simulink model "a4"  (R2018b)
settings: Solver=ode23tb  StartTime=0.0  StopTime=24*60*60  MaxStep=60  RelTol=1e-4
PreLoadFcn:
  | load('solar_load_data_24h.mat')
(part 2 of 2)

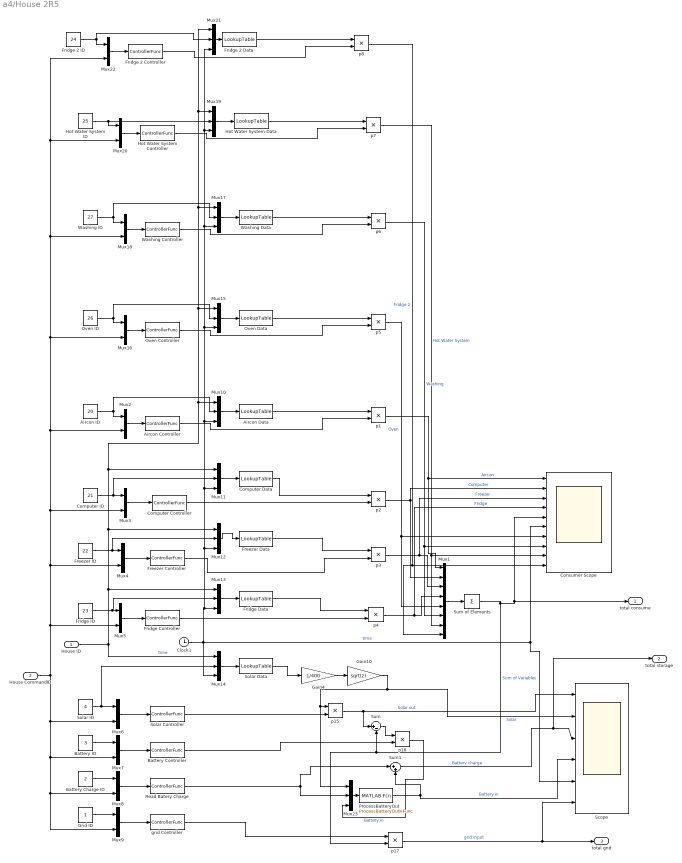
== system a4/House 2R5 ==
  House ID : Inport
  House CommandID : Inport  Port=2
  Aircon Controller : MATLABFcn  MATLABFcn=ControllerFunc  OutputSignalType=real
  Aircon Data : MATLABFcn  MATLABFcn=LookupTable  OutputSignalType=real
  Aircon ID : Constant  Value=20
  Battery Charge ID : Constant  Value=2
  Battery Controller : MATLABFcn  MATLABFcn=ControllerFunc  OutputSignalType=real
  Battery ID : Constant  Value=3
  Clock1 : Clock
  Computer Controller : MATLABFcn  MATLABFcn=ControllerFunc  OutputSignalType=real
  Computer Data : MATLABFcn  MATLABFcn=LookupTable  OutputSignalType=real
  Computer ID : Constant  Value=21
  Consumer Scope : Scope  NumInputPorts=10
  Freezer Controller : MATLABFcn  MATLABFcn=ControllerFunc  OutputSignalType=real
  Freezer Data : MATLABFcn  MATLABFcn=LookupTable  OutputSignalType=real
  Freezer ID : Constant  Value=22
  Fridge 2 Controller : MATLABFcn  MATLABFcn=ControllerFunc  OutputSignalType=real
  Fridge 2 Data : MATLABFcn  MATLABFcn=LookupTable  OutputSignalType=real
  Fridge 2 ID : Constant  Value=24
  Fridge Controller : MATLABFcn  MATLABFcn=ControllerFunc  OutputSignalType=real
  Fridge Data : MATLABFcn  MATLABFcn=LookupTable  OutputSignalType=real
  Fridge ID : Constant  Value=23
  Gain10 : Gain  Gain=sqrt(2)
  Gain4 : Gain  Gain=1/400
  Grid ID : Constant
  Hot Water System Controller : MATLABFcn  MATLABFcn=ControllerFunc  OutputSignalType=real
  Hot Water System Data : MATLABFcn  MATLABFcn=LookupTable  OutputSignalType=real
  Hot Water System ID : Constant  Value=25
  Mux1 : Mux  Inputs=8
  Mux{10..15,17,19,21,23} (10 alike) : Mux  Inputs=3
  Mux{2..9,16,18,20,22} (12 alike) : Mux  Inputs=2
  Oven Controller : MATLABFcn  MATLABFcn=ControllerFunc  OutputSignalType=real
  Oven Data : MATLABFcn  MATLABFcn=LookupTable  OutputSignalType=real
  Oven ID : Constant  Value=26
  ProcessBatteryOut : MATLABFcn  MATLABFcn=ProcessBatteryOutHFunc  OutputSignalType=real
  Read Batery Charge : MATLABFcn  MATLABFcn=ControllerFunc  OutputSignalType=real
  Scope : Scope  NumInputPorts=6
  Solar Controller : MATLABFcn  MATLABFcn=ControllerFunc  OutputSignalType=real
  Solar Data : MATLABFcn  MATLABFcn=LookupTable  OutputSignalType=real
  Solar ID : Constant  Value=4
  Sum : Sum  Inputs=|+-
  Sum of Elements : Sum  Inputs=+
  Sum1 : Sum  Inputs=|++
  Washing Controller : MATLABFcn  MATLABFcn=ControllerFunc  OutputSignalType=real
  Washing Data : MATLABFcn  MATLABFcn=LookupTable  OutputSignalType=real
  Washing ID : Constant  Value=27
  grid Controller : MATLABFcn  MATLABFcn=ControllerFunc  OutputSignalType=real
  p{1..8,15..17} (11 alike) : Product
  total consume : Outport
  total storage : Outport  Port=2
  total grid : Outport  Port=3
  wires:
  Clock1/1 -> Mux11/3, Mux21/3, Mux19/3, Mux17/3, Mux15/3, Mux10/3, Mux12/3, Mux13/3, Mux14/3, Scope/5, Consumer Scope/6  "time"
  Aircon Data/1 -> p1/1
  Mux1/1 -> Sum of Elements/1
  p1/1 -> Consumer Scope/1, Mux1/1  "Aircon"
  Sum of Elements/1 -> total consume/1, Consumer Scope/5, p17/2, Sum/2  "Sum of Variables"
  p4/1 -> Consumer Scope/4, Mux1/4  "Fridge"
  p2/1 -> Consumer Scope/2, Mux1/2  "Computer"
  p3/1 -> Consumer Scope/3, Mux1/3  "Freezer"
  Computer Controller/1 -> p2/2
  Freezer Controller/1 -> p3/2
  Solar Data/1 -> Gain4/1
  Solar Controller/1 -> p15/2
  Gain10/1 -> Scope/2, Mux23/1, p15/1  "Solar"
  p15/1 -> Sum/1, Scope/1  "Solar out"
  Sum/1 -> p16/1
  Battery Controller/1 -> p16/2
  Sum1/1 -> total storage/1, Scope/3  "Battery charge"
  grid Controller/1 -> p17/1
  p17/1 -> Scope/6, total grid/1  "grid input"
  Read Batery Charge/1 -> Mux23/2, Sum1/1
  p16/1 -> Mux23/3  "Battery in"
  ProcessBatteryOut/1 -> Scope/4, Sum1/2  "Battery in"
  Computer Data/1 -> p2/1
  Freezer Data/1 -> p3/1
  Fridge Data/1 -> p4/1
  Fridge Controller/1 -> p4/2
  Gain4/1 -> Gain10/1
  Aircon ID/1 -> Mux2/1, Mux10/2
  Computer ID/1 -> Mux11/2, Mux3/1
  Mux3/1 -> Computer Controller/1
  Freezer ID/1 -> Mux12/2, Mux4/1
  Mux4/1 -> Freezer Controller/1
  Mux5/1 -> Fridge Controller/1
  Fridge ID/1 -> Mux13/2, Mux5/1
  Mux6/1 -> Solar Controller/1
  Solar ID/1 -> Mux14/2, Mux6/1
  Mux7/1 -> Battery Controller/1
  Mux8/1 -> Read Batery Charge/1
  Mux9/1 -> grid Controller/1
  Battery ID/1 -> Mux7/1
  Battery Charge ID/1 -> Mux8/1
  Grid ID/1 -> Mux9/1
  Mux10/1 -> Aircon Data/1
  Mux11/1 -> Computer Data/1
  Mux12/1 -> Freezer Data/1
  Mux13/1 -> Fridge Data/1
  Mux14/1 -> Solar Data/1
  Aircon Controller/1 -> p1/2
  Mux2/1 -> Aircon Controller/1
  House CommandID/1 -> Mux9/2, Mux8/2, Mux7/2, Mux6/2, Mux3/2, Mux16/2, Mux20/2, Mux22/2, Mux18/2, Mux2/2, Mux4/2, Mux5/2
  Oven Data/1 -> p5/1
  Oven ID/1 -> Mux16/1, Mux15/2
  Mux15/1 -> Oven Data/1
  p5/1 -> Mux1/5, Consumer Scope/7  "Oven"
  Oven Controller/1 -> p5/2
  Washing Data/1 -> p6/1
  Washing ID/1 -> Mux18/1, Mux17/2
  Mux17/1 -> Washing Data/1
  p6/1 -> Mux1/6, Consumer Scope/8  "Washing"
  Washing Controller/1 -> p6/2
  Hot Water System Data/1 -> p7/1
  Hot Water System ID/1 -> Mux20/1, Mux19/2
  Mux19/1 -> Hot Water System Data/1
  p7/1 -> Mux1/7, Consumer Scope/9  "Hot Water System"
  Hot Water System Controller/1 -> p7/2
  Fridge 2 Data/1 -> p8/1
  Fridge 2 ID/1 -> Mux22/1, Mux21/2
  Mux21/1 -> Fridge 2 Data/1
  p8/1 -> Consumer Scope/10, Mux1/8  "Fridge 2"
  Fridge 2 Controller/1 -> p8/2
  House ID/1 -> Mux14/1, Mux21/1, Mux19/1, Mux17/1, Mux15/1, Mux10/1, Mux11/1, Mux12/1, Mux13/1  "time"
  Mux20/1 -> Hot Water System Controller/1
  Mux16/1 -> Oven Controller/1
  Mux18/1 -> Washing Controller/1
  Mux22/1 -> Fridge 2 Controller/1
  Mux23/1 -> ProcessBatteryOut/1

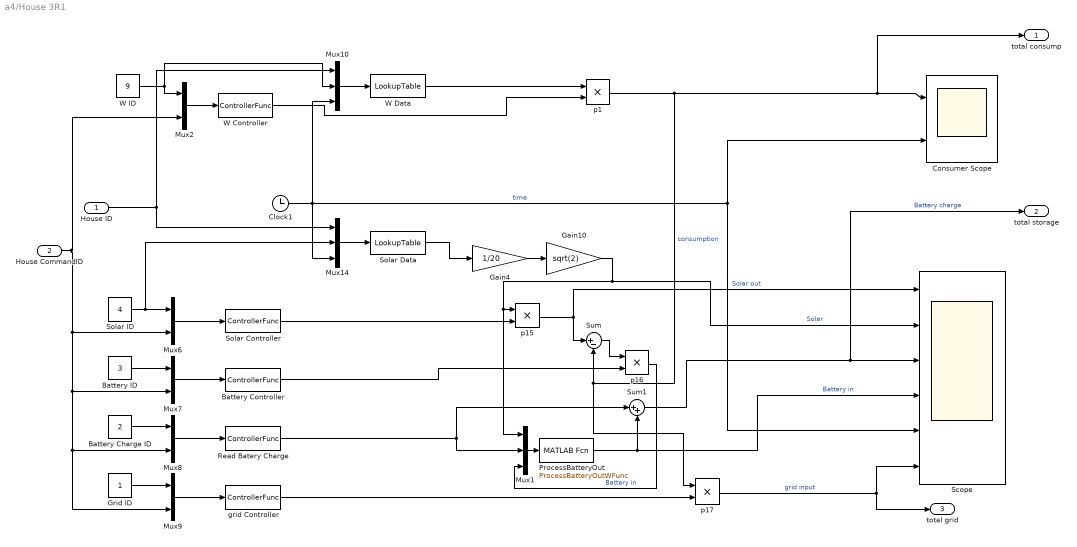
== system a4/House 3R1 ==
  House ID : Inport
  House CommandID : Inport  Port=2
  Battery Charge ID : Constant  Value=2
  Battery Controller : MATLABFcn  MATLABFcn=ControllerFunc  OutputSignalType=real
  Battery ID : Constant  Value=3
  Clock1 : Clock
  Consumer Scope : Scope  NumInputPorts=2
  Gain10 : Gain  Gain=sqrt(2)
  Gain4 : Gain  Gain=1/20
  Grid ID : Constant
  Mux1 : Mux  Inputs=3
  Mux10 : Mux  Inputs=3
  Mux14 : Mux  Inputs=3
  Mux{2,6..9} (5 alike) : Mux  Inputs=2
  ProcessBatteryOut : MATLABFcn  MATLABFcn=ProcessBatteryOutWFunc  OutputSignalType=real
  Read Batery Charge : MATLABFcn  MATLABFcn=ControllerFunc  OutputSignalType=real
  Scope : Scope  NumInputPorts=6
  Solar Controller : MATLABFcn  MATLABFcn=ControllerFunc  OutputSignalType=real
  Solar Data : MATLABFcn  MATLABFcn=LookupTable  OutputSignalType=real
  Solar ID : Constant  Value=4
  Sum : Sum  Inputs=|+-
  Sum1 : Sum  Inputs=|++
  W Controller : MATLABFcn  MATLABFcn=ControllerFunc  OutputSignalType=real
  W Data : MATLABFcn  MATLABFcn=LookupTable  OutputSignalType=real
  W ID : Constant  Value=9
  grid Controller : MATLABFcn  MATLABFcn=ControllerFunc  OutputSignalType=real
  p{1,15..17} (4 alike) : Product
  total consump : Outport
  total storage : Outport  Port=2
  total grid : Outport  Port=3
  wires:
  Clock1/1 -> Mux10/3, Mux14/3, Scope/5, Consumer Scope/2  "time"
  W Data/1 -> p1/1
  Solar Data/1 -> Gain4/1
  Solar Controller/1 -> p15/2
  Gain10/1 -> Scope/2, Mux1/1, p15/1  "Solar"
  p15/1 -> Sum/1, Scope/1  "Solar out"
  Sum/1 -> p16/1
  Battery Controller/1 -> p16/2
  Sum1/1 -> total storage/1, Scope/3  "Battery charge"
  grid Controller/1 -> p17/2
  p17/1 -> Scope/6, total grid/1  "grid input"
  Read Batery Charge/1 -> Sum1/1, Mux1/2
  p16/1 -> Mux1/3  "Battery in"
  ProcessBatteryOut/1 -> Scope/4, Sum1/2  "Battery in"
  Mux1/1 -> ProcessBatteryOut/1
  Gain4/1 -> Gain10/1
  W ID/1 -> Mux2/1, Mux10/2
  House ID/1 -> Mux10/1, Mux14/1
  Mux6/1 -> Solar Controller/1
  Solar ID/1 -> Mux14/2, Mux6/1
  Mux7/1 -> Battery Controller/1
  Mux8/1 -> Read Batery Charge/1
  Mux9/1 -> grid Controller/1
  Battery ID/1 -> Mux7/1
  Battery Charge ID/1 -> Mux8/1
  Grid ID/1 -> Mux9/1
  Mux10/1 -> W Data/1
  Mux14/1 -> Solar Data/1
  W Controller/1 -> p1/2
  Mux2/1 -> W Controller/1
  p1/1 -> p17/1, Sum/2, total consump/1, Consumer Scope/1  "consumption"
  House CommandID/1 -> Mux9/2, Mux8/2, Mux7/2, Mux6/2, Mux2/2

== system a4/House 3R2 ==
  House ID : Inport
  House CommandID : Inport  Port=2
  Battery Charge ID : Constant  Value=2
  Battery Controller : MATLABFcn  MATLABFcn=ControllerFunc  OutputSignalType=real
  Battery ID : Constant  Value=3
  Clock1 : Clock
  Consumer Scope : Scope  NumInputPorts=2
  Gain10 : Gain  Gain=sqrt(2)
  Gain4 : Gain  Gain=1/20
  Grid ID : Constant
  Mux1 : Mux  Inputs=3
  Mux10 : Mux  Inputs=3
  Mux14 : Mux  Inputs=3
  Mux{2,6..9} (5 alike) : Mux  Inputs=2
  ProcessBatteryOut : MATLABFcn  MATLABFcn=ProcessBatteryOutWFunc  OutputSignalType=real
  Read Batery Charge : MATLABFcn  MATLABFcn=ControllerFunc  OutputSignalType=real
  Scope : Scope  NumInputPorts=6
  Solar Controller : MATLABFcn  MATLABFcn=ControllerFunc  OutputSignalType=real
  Solar Data : MATLABFcn  MATLABFcn=LookupTable  OutputSignalType=real
  Solar ID : Constant  Value=4
  Sum : Sum  Inputs=|+-
  Sum1 : Sum  Inputs=|++
  W Controller : MATLABFcn  MATLABFcn=ControllerFunc  OutputSignalType=real
  W Data : MATLABFcn  MATLABFcn=LookupTable  OutputSignalType=real
  W ID : Constant  Value=9
  grid Controller : MATLABFcn  MATLABFcn=ControllerFunc  OutputSignalType=real
  p{1,15..17} (4 alike) : Product
  total consump : Outport
  total storage : Outport  Port=2
  total grid : Outport  Port=3
  wires:
  House CommandID/1 -> Mux2/2, Mux6/2, Mux7/2, Mux8/2, Mux9/2
  p1/1 -> Consumer Scope/1, total consump/1, Sum/2, p17/1  "consumption"
  Mux2/1 -> W Controller/1
  W Controller/1 -> p1/2
  Mux14/1 -> Solar Data/1
  Mux10/1 -> W Data/1
  Grid ID/1 -> Mux9/1
  Battery Charge ID/1 -> Mux8/1
  Battery ID/1 -> Mux7/1
  Mux9/1 -> grid Controller/1
  Mux8/1 -> Read Batery Charge/1
  Mux7/1 -> Battery Controller/1
  Solar ID/1 -> Mux6/1, Mux14/2
  Mux6/1 -> Solar Controller/1
  House ID/1 -> Mux14/1, Mux10/1
  W ID/1 -> Mux10/2, Mux2/1
  Gain4/1 -> Gain10/1
  Mux1/1 -> ProcessBatteryOut/1
  ProcessBatteryOut/1 -> Sum1/2, Scope/4  "Battery in"
  p16/1 -> Mux1/3  "Battery in"
  Read Batery Charge/1 -> Mux1/2, Sum1/1
  p17/1 -> total grid/1, Scope/6  "grid input"
  grid Controller/1 -> p17/2
  Sum1/1 -> Scope/3, total storage/1  "Battery charge"
  Battery Controller/1 -> p16/2
  Sum/1 -> p16/1
  p15/1 -> Scope/1, Sum/1  "Solar out"
  Gain10/1 -> p15/1, Mux1/1, Scope/2  "Solar"
  Solar Controller/1 -> p15/2
  Solar Data/1 -> Gain4/1
  W Data/1 -> p1/1
  Clock1/1 -> Consumer Scope/2, Scope/5, Mux14/3, Mux10/3  "time"

== system a4/House 3R3 ==
  House ID : Inport
  House CommandID : Inport  Port=2
  Battery Charge ID : Constant  Value=2
  Battery Controller : MATLABFcn  MATLABFcn=ControllerFunc  OutputSignalType=real
  Battery ID : Constant  Value=3
  Clock1 : Clock
  Consumer Scope : Scope  NumInputPorts=2
  Gain10 : Gain  Gain=sqrt(2)
  Gain4 : Gain  Gain=1/20
  Grid ID : Constant
  Mux1 : Mux  Inputs=3
  Mux10 : Mux  Inputs=3
  Mux14 : Mux  Inputs=3
  Mux{2,6..9} (5 alike) : Mux  Inputs=2
  ProcessBatteryOut : MATLABFcn  MATLABFcn=ProcessBatteryOutWFunc  OutputSignalType=real
  Read Batery Charge : MATLABFcn  MATLABFcn=ControllerFunc  OutputSignalType=real
  Scope : Scope  NumInputPorts=6
  Solar Controller : MATLABFcn  MATLABFcn=ControllerFunc  OutputSignalType=real
  Solar Data : MATLABFcn  MATLABFcn=LookupTable  OutputSignalType=real
  Solar ID : Constant  Value=4
  Sum : Sum  Inputs=|+-
  Sum1 : Sum  Inputs=|++
  W Controller : MATLABFcn  MATLABFcn=ControllerFunc  OutputSignalType=real
  W Data : MATLABFcn  MATLABFcn=LookupTable  OutputSignalType=real
  W ID : Constant  Value=9
  grid Controller : MATLABFcn  MATLABFcn=ControllerFunc  OutputSignalType=real
  p{1,15..17} (4 alike) : Product
  total consump : Outport
  total storage : Outport  Port=2
  total grid : Outport  Port=3
  wires:
  Clock1/1 -> Mux10/3, Mux14/3, Scope/5, Consumer Scope/2  "time"
  W Data/1 -> p1/1
  Solar Data/1 -> Gain4/1
  Solar Controller/1 -> p15/2
  Gain10/1 -> Scope/2, Mux1/1, p15/1  "Solar"
  p15/1 -> Sum/1, Scope/1  "Solar out"
  Sum/1 -> p16/1
  Battery Controller/1 -> p16/2
  Sum1/1 -> total storage/1, Scope/3  "Battery charge"
  grid Controller/1 -> p17/2
  p17/1 -> Scope/6, total grid/1  "grid input"
  Read Batery Charge/1 -> Sum1/1, Mux1/2
  p16/1 -> Mux1/3  "Battery in"
  ProcessBatteryOut/1 -> Scope/4, Sum1/2  "Battery in"
  Mux1/1 -> ProcessBatteryOut/1
  Gain4/1 -> Gain10/1
  W ID/1 -> Mux2/1, Mux10/2
  House ID/1 -> Mux10/1, Mux14/1
  Mux6/1 -> Solar Controller/1
  Solar ID/1 -> Mux14/2, Mux6/1
  Mux7/1 -> Battery Controller/1
  Mux8/1 -> Read Batery Charge/1
  Mux9/1 -> grid Controller/1
  Battery ID/1 -> Mux7/1
  Battery Charge ID/1 -> Mux8/1
  Grid ID/1 -> Mux9/1
  Mux10/1 -> W Data/1
  Mux14/1 -> Solar Data/1
  W Controller/1 -> p1/2
  Mux2/1 -> W Controller/1
  p1/1 -> p17/1, Sum/2, total consump/1, Consumer Scope/1  "consumption"
  House CommandID/1 -> Mux9/2, Mux8/2, Mux7/2, Mux6/2, Mux2/2

== system a4/House 3R4 ==
  House ID : Inport
  House CommandID : Inport  Port=2
  Battery Charge ID : Constant  Value=2
  Battery Controller : MATLABFcn  MATLABFcn=ControllerFunc  OutputSignalType=real
  Battery ID : Constant  Value=3
  Clock1 : Clock
  Consumer Scope : Scope  NumInputPorts=2
  Gain10 : Gain  Gain=sqrt(2)
  Gain4 : Gain  Gain=1/20
  Grid ID : Constant
  Mux1 : Mux  Inputs=3
  Mux10 : Mux  Inputs=3
  Mux14 : Mux  Inputs=3
  Mux{2,6..9} (5 alike) : Mux  Inputs=2
  ProcessBatteryOut : MATLABFcn  MATLABFcn=ProcessBatteryOutWFunc  OutputSignalType=real
  Read Batery Charge : MATLABFcn  MATLABFcn=ControllerFunc  OutputSignalType=real
  Scope : Scope  NumInputPorts=6
  Solar Controller : MATLABFcn  MATLABFcn=ControllerFunc  OutputSignalType=real
  Solar Data : MATLABFcn  MATLABFcn=LookupTable  OutputSignalType=real
  Solar ID : Constant  Value=4
  Sum : Sum  Inputs=|+-
  Sum1 : Sum  Inputs=|++
  W Controller : MATLABFcn  MATLABFcn=ControllerFunc  OutputSignalType=real
  W Data : MATLABFcn  MATLABFcn=LookupTable  OutputSignalType=real
  W ID : Constant  Value=9
  grid Controller : MATLABFcn  MATLABFcn=ControllerFunc  OutputSignalType=real
  p{1,15..17} (4 alike) : Product
  total consump : Outport
  total storage : Outport  Port=2
  total grid : Outport  Port=3
  wires:
  House CommandID/1 -> Mux2/2, Mux6/2, Mux7/2, Mux8/2, Mux9/2
  p1/1 -> Consumer Scope/1, total consump/1, Sum/2, p17/1  "consumption"
  Mux2/1 -> W Controller/1
  W Controller/1 -> p1/2
  Mux14/1 -> Solar Data/1
  Mux10/1 -> W Data/1
  Grid ID/1 -> Mux9/1
  Battery Charge ID/1 -> Mux8/1
  Battery ID/1 -> Mux7/1
  Mux9/1 -> grid Controller/1
  Mux8/1 -> Read Batery Charge/1
  Mux7/1 -> Battery Controller/1
  Solar ID/1 -> Mux6/1, Mux14/2
  Mux6/1 -> Solar Controller/1
  House ID/1 -> Mux14/1, Mux10/1
  W ID/1 -> Mux10/2, Mux2/1
  Gain4/1 -> Gain10/1
  Mux1/1 -> ProcessBatteryOut/1
  ProcessBatteryOut/1 -> Sum1/2, Scope/4  "Battery in"
  p16/1 -> Mux1/3  "Battery in"
  Read Batery Charge/1 -> Mux1/2, Sum1/1
  p17/1 -> total grid/1, Scope/6  "grid input"
  grid Controller/1 -> p17/2
  Sum1/1 -> Scope/3, total storage/1  "Battery charge"
  Battery Controller/1 -> p16/2
  Sum/1 -> p16/1
  p15/1 -> Scope/1, Sum/1  "Solar out"
  Gain10/1 -> p15/1, Mux1/1, Scope/2  "Solar"
  Solar Controller/1 -> p15/2
  Solar Data/1 -> Gain4/1
  W Data/1 -> p1/1
  Clock1/1 -> Consumer Scope/2, Scope/5, Mux14/3, Mux10/3  "time"

== system a4/House 3R5 ==
  House ID : Inport
  House CommandID : Inport  Port=2
  Battery Charge ID : Constant  Value=2
  Battery Controller : MATLABFcn  MATLABFcn=ControllerFunc  OutputSignalType=real
  Battery ID : Constant  Value=3
  Clock1 : Clock
  Consumer Scope : Scope  NumInputPorts=2
  Gain10 : Gain  Gain=sqrt(2)
  Gain4 : Gain  Gain=1/20
  Grid ID : Constant
  Mux1 : Mux  Inputs=3
  Mux10 : Mux  Inputs=3
  Mux14 : Mux  Inputs=3
  Mux{2,6..9} (5 alike) : Mux  Inputs=2
  ProcessBatteryOut : MATLABFcn  MATLABFcn=ProcessBatteryOutWFunc  OutputSignalType=real
  Read Batery Charge : MATLABFcn  MATLABFcn=ControllerFunc  OutputSignalType=real
  Scope : Scope  NumInputPorts=6
  Solar Controller : MATLABFcn  MATLABFcn=ControllerFunc  OutputSignalType=real
  Solar Data : MATLABFcn  MATLABFcn=LookupTable  OutputSignalType=real
  Solar ID : Constant  Value=4
  Sum : Sum  Inputs=|+-
  Sum1 : Sum  Inputs=|++
  W Controller : MATLABFcn  MATLABFcn=ControllerFunc  OutputSignalType=real
  W Data : MATLABFcn  MATLABFcn=LookupTable  OutputSignalType=real
  W ID : Constant  Value=9
  grid Controller : MATLABFcn  MATLABFcn=ControllerFunc  OutputSignalType=real
  p{1,15..17} (4 alike) : Product
  total consump : Outport
  total storage : Outport  Port=2
  total grid : Outport  Port=3
  wires:
  Clock1/1 -> Mux10/3, Mux14/3, Scope/5, Consumer Scope/2  "time"
  W Data/1 -> p1/1
  Solar Data/1 -> Gain4/1
  Solar Controller/1 -> p15/2
  Gain10/1 -> Scope/2, Mux1/1, p15/1  "Solar"
  p15/1 -> Sum/1, Scope/1  "Solar out"
  Sum/1 -> p16/1
  Battery Controller/1 -> p16/2
  Sum1/1 -> total storage/1, Scope/3  "Battery charge"
  grid Controller/1 -> p17/2
  p17/1 -> Scope/6, total grid/1  "grid input"
  Read Batery Charge/1 -> Sum1/1, Mux1/2
  p16/1 -> Mux1/3  "Battery in"
  ProcessBatteryOut/1 -> Scope/4, Sum1/2  "Battery in"
  Mux1/1 -> ProcessBatteryOut/1
  Gain4/1 -> Gain10/1
  W ID/1 -> Mux2/1, Mux10/2
  House ID/1 -> Mux10/1, Mux14/1
  Mux6/1 -> Solar Controller/1
  Solar ID/1 -> Mux14/2, Mux6/1
  Mux7/1 -> Battery Controller/1
  Mux8/1 -> Read Batery Charge/1
  Mux9/1 -> grid Controller/1
  Battery ID/1 -> Mux7/1
  Battery Charge ID/1 -> Mux8/1
  Grid ID/1 -> Mux9/1
  Mux10/1 -> W Data/1
  Mux14/1 -> Solar Data/1
  W Controller/1 -> p1/2
  Mux2/1 -> W Controller/1
  p1/1 -> p17/1, Sum/2, total consump/1, Consumer Scope/1  "consumption"
  House CommandID/1 -> Mux9/2, Mux8/2, Mux7/2, Mux6/2, Mux2/2

== system a4/House 4R1 ==
  House ID : Inport
  House CommandID : Inport  Port=2
  Battery Charge ID : Constant  Value=2
  Battery Controller : MATLABFcn  MATLABFcn=ControllerFunc  OutputSignalType=real
  Battery ID : Constant  Value=3
  Clock1 : Clock
  Consumer Scope : Scope  NumInputPorts=2
  Gain10 : Gain  Gain=sqrt(2)
  Gain4 : Gain  Gain=1/20
  Grid ID : Constant
  Mux1 : Mux  Inputs=3
  Mux10 : Mux  Inputs=3
  Mux14 : Mux  Inputs=3
  Mux{2,6..9} (5 alike) : Mux  Inputs=2
  ProcessBatteryOut : MATLABFcn  MATLABFcn=ProcessBatteryOutWFunc  OutputSignalType=real
  Read Batery Charge : MATLABFcn  MATLABFcn=ControllerFunc  OutputSignalType=real
  Scope : Scope  NumInputPorts=6
  Solar Controller : MATLABFcn  MATLABFcn=ControllerFunc  OutputSignalType=real
  Solar Data : MATLABFcn  MATLABFcn=LookupTable  OutputSignalType=real
  Solar ID : Constant  Value=4
  Sum : Sum  Inputs=|+-
  Sum1 : Sum  Inputs=|++
  W Controller : MATLABFcn  MATLABFcn=ControllerFunc  OutputSignalType=real
  W Data : MATLABFcn  MATLABFcn=LookupTable  OutputSignalType=real
  W ID : Constant  Value=9
  grid Controller : MATLABFcn  MATLABFcn=ControllerFunc  OutputSignalType=real
  p{1,15..17} (4 alike) : Product
  total consump : Outport
  total storage : Outport  Port=2
  total grid : Outport  Port=3
  wires:
  House CommandID/1 -> Mux2/2, Mux6/2, Mux7/2, Mux8/2, Mux9/2
  p1/1 -> Consumer Scope/1, total consump/1, Sum/2, p17/1  "consumption"
  Mux2/1 -> W Controller/1
  W Controller/1 -> p1/2
  Mux14/1 -> Solar Data/1
  Mux10/1 -> W Data/1
  Grid ID/1 -> Mux9/1
  Battery Charge ID/1 -> Mux8/1
  Battery ID/1 -> Mux7/1
  Mux9/1 -> grid Controller/1
  Mux8/1 -> Read Batery Charge/1
  Mux7/1 -> Battery Controller/1
  Solar ID/1 -> Mux6/1, Mux14/2
  Mux6/1 -> Solar Controller/1
  House ID/1 -> Mux14/1, Mux10/1
  W ID/1 -> Mux10/2, Mux2/1
  Gain4/1 -> Gain10/1
  Mux1/1 -> ProcessBatteryOut/1
  ProcessBatteryOut/1 -> Sum1/2, Scope/4  "Battery in"
  p16/1 -> Mux1/3  "Battery in"
  Read Batery Charge/1 -> Mux1/2, Sum1/1
  p17/1 -> total grid/1, Scope/6  "grid input"
  grid Controller/1 -> p17/2
  Sum1/1 -> Scope/3, total storage/1  "Battery charge"
  Battery Controller/1 -> p16/2
  Sum/1 -> p16/1
  p15/1 -> Scope/1, Sum/1  "Solar out"
  Gain10/1 -> p15/1, Mux1/1, Scope/2  "Solar"
  Solar Controller/1 -> p15/2
  Solar Data/1 -> Gain4/1
  W Data/1 -> p1/1
  Clock1/1 -> Consumer Scope/2, Scope/5, Mux14/3, Mux10/3  "time"

== system a4/House 4R2 ==
  House ID : Inport
  House CommandID : Inport  Port=2
  Battery Charge ID : Constant  Value=2
  Battery Controller : MATLABFcn  MATLABFcn=ControllerFunc  OutputSignalType=real
  Battery ID : Constant  Value=3
  Clock1 : Clock
  Consumer Scope : Scope  NumInputPorts=2
  Gain10 : Gain  Gain=sqrt(2)
  Gain4 : Gain  Gain=1/20
  Grid ID : Constant
  Mux1 : Mux  Inputs=3
  Mux10 : Mux  Inputs=3
  Mux14 : Mux  Inputs=3
  Mux{2,6..9} (5 alike) : Mux  Inputs=2
  ProcessBatteryOut : MATLABFcn  MATLABFcn=ProcessBatteryOutWFunc  OutputSignalType=real
  Read Batery Charge : MATLABFcn  MATLABFcn=ControllerFunc  OutputSignalType=real
  Scope : Scope  NumInputPorts=6
  Solar Controller : MATLABFcn  MATLABFcn=ControllerFunc  OutputSignalType=real
  Solar Data : MATLABFcn  MATLABFcn=LookupTable  OutputSignalType=real
  Solar ID : Constant  Value=4
  Sum : Sum  Inputs=|+-
  Sum1 : Sum  Inputs=|++
  W Controller : MATLABFcn  MATLABFcn=ControllerFunc  OutputSignalType=real
  W Data : MATLABFcn  MATLABFcn=LookupTable  OutputSignalType=real
  W ID : Constant  Value=9
  grid Controller : MATLABFcn  MATLABFcn=ControllerFunc  OutputSignalType=real
  p{1,15..17} (4 alike) : Product
  total consump : Outport
  total storage : Outport  Port=2
  total grid : Outport  Port=3
  wires:
  Clock1/1 -> Mux10/3, Mux14/3, Scope/5, Consumer Scope/2  "time"
  W Data/1 -> p1/1
  Solar Data/1 -> Gain4/1
  Solar Controller/1 -> p15/2
  Gain10/1 -> Scope/2, Mux1/1, p15/1  "Solar"
  p15/1 -> Sum/1, Scope/1  "Solar out"
  Sum/1 -> p16/1
  Battery Controller/1 -> p16/2
  Sum1/1 -> total storage/1, Scope/3  "Battery charge"
  grid Controller/1 -> p17/2
  p17/1 -> Scope/6, total grid/1  "grid input"
  Read Batery Charge/1 -> Sum1/1, Mux1/2
  p16/1 -> Mux1/3  "Battery in"
  ProcessBatteryOut/1 -> Scope/4, Sum1/2  "Battery in"
  Mux1/1 -> ProcessBatteryOut/1
  Gain4/1 -> Gain10/1
  W ID/1 -> Mux2/1, Mux10/2
  House ID/1 -> Mux10/1, Mux14/1
  Mux6/1 -> Solar Controller/1
  Solar ID/1 -> Mux14/2, Mux6/1
  Mux7/1 -> Battery Controller/1
  Mux8/1 -> Read Batery Charge/1
  Mux9/1 -> grid Controller/1
  Battery ID/1 -> Mux7/1
  Battery Charge ID/1 -> Mux8/1
  Grid ID/1 -> Mux9/1
  Mux10/1 -> W Data/1
  Mux14/1 -> Solar Data/1
  W Controller/1 -> p1/2
  Mux2/1 -> W Controller/1
  p1/1 -> p17/1, Sum/2, total consump/1, Consumer Scope/1  "consumption"
  House CommandID/1 -> Mux9/2, Mux8/2, Mux7/2, Mux6/2, Mux2/2

== system a4/House 4R3 ==
  House ID : Inport
  House CommandID : Inport  Port=2
  Battery Charge ID : Constant  Value=2
  Battery Controller : MATLABFcn  MATLABFcn=ControllerFunc  OutputSignalType=real
  Battery ID : Constant  Value=3
  Clock1 : Clock
  Consumer Scope : Scope  NumInputPorts=2
  Gain10 : Gain  Gain=sqrt(2)
  Gain4 : Gain  Gain=1/20
  Grid ID : Constant
  Mux1 : Mux  Inputs=3
  Mux10 : Mux  Inputs=3
  Mux14 : Mux  Inputs=3
  Mux{2,6..9} (5 alike) : Mux  Inputs=2
  ProcessBatteryOut : MATLABFcn  MATLABFcn=ProcessBatteryOutWFunc  OutputSignalType=real
  Read Batery Charge : MATLABFcn  MATLABFcn=ControllerFunc  OutputSignalType=real
  Scope : Scope  NumInputPorts=6
  Solar Controller : MATLABFcn  MATLABFcn=ControllerFunc  OutputSignalType=real
  Solar Data : MATLABFcn  MATLABFcn=LookupTable  OutputSignalType=real
  Solar ID : Constant  Value=4
  Sum : Sum  Inputs=|+-
  Sum1 : Sum  Inputs=|++
  W Controller : MATLABFcn  MATLABFcn=ControllerFunc  OutputSignalType=real
  W Data : MATLABFcn  MATLABFcn=LookupTable  OutputSignalType=real
  W ID : Constant  Value=9
  grid Controller : MATLABFcn  MATLABFcn=ControllerFunc  OutputSignalType=real
  p{1,15..17} (4 alike) : Product
  total consump : Outport
  total storage : Outport  Port=2
  total grid : Outport  Port=3
  wires:
  House CommandID/1 -> Mux2/2, Mux6/2, Mux7/2, Mux8/2, Mux9/2
  p1/1 -> Consumer Scope/1, total consump/1, Sum/2, p17/1  "consumption"
  Mux2/1 -> W Controller/1
  W Controller/1 -> p1/2
  Mux14/1 -> Solar Data/1
  Mux10/1 -> W Data/1
  Grid ID/1 -> Mux9/1
  Battery Charge ID/1 -> Mux8/1
  Battery ID/1 -> Mux7/1
  Mux9/1 -> grid Controller/1
  Mux8/1 -> Read Batery Charge/1
  Mux7/1 -> Battery Controller/1
  Solar ID/1 -> Mux6/1, Mux14/2
  Mux6/1 -> Solar Controller/1
  House ID/1 -> Mux14/1, Mux10/1
  W ID/1 -> Mux10/2, Mux2/1
  Gain4/1 -> Gain10/1
  Mux1/1 -> ProcessBatteryOut/1
  ProcessBatteryOut/1 -> Sum1/2, Scope/4  "Battery in"
  p16/1 -> Mux1/3  "Battery in"
  Read Batery Charge/1 -> Mux1/2, Sum1/1
  p17/1 -> total grid/1, Scope/6  "grid input"
  grid Controller/1 -> p17/2
  Sum1/1 -> Scope/3, total storage/1  "Battery charge"
  Battery Controller/1 -> p16/2
  Sum/1 -> p16/1
  p15/1 -> Scope/1, Sum/1  "Solar out"
  Gain10/1 -> p15/1, Mux1/1, Scope/2  "Solar"
  Solar Controller/1 -> p15/2
  Solar Data/1 -> Gain4/1
  W Data/1 -> p1/1
  Clock1/1 -> Consumer Scope/2, Scope/5, Mux14/3, Mux10/3  "time"

== system a4/House 4R4 ==
  House ID : Inport
  House CommandID : Inport  Port=2
  Battery Charge ID : Constant  Value=2
  Battery Controller : MATLABFcn  MATLABFcn=ControllerFunc  OutputSignalType=real
  Battery ID : Constant  Value=3
  Clock1 : Clock
  Consumer Scope : Scope  NumInputPorts=2
  Gain10 : Gain  Gain=sqrt(2)
  Gain4 : Gain  Gain=1/20
  Grid ID : Constant
  Mux1 : Mux  Inputs=3
  Mux10 : Mux  Inputs=3
  Mux14 : Mux  Inputs=3
  Mux{2,6..9} (5 alike) : Mux  Inputs=2
  ProcessBatteryOut : MATLABFcn  MATLABFcn=ProcessBatteryOutWFunc  OutputSignalType=real
  Read Batery Charge : MATLABFcn  MATLABFcn=ControllerFunc  OutputSignalType=real
  Scope : Scope  NumInputPorts=6
  Solar Controller : MATLABFcn  MATLABFcn=ControllerFunc  OutputSignalType=real
  Solar Data : MATLABFcn  MATLABFcn=LookupTable  OutputSignalType=real
  Solar ID : Constant  Value=4
  Sum : Sum  Inputs=|+-
  Sum1 : Sum  Inputs=|++
  W Controller : MATLABFcn  MATLABFcn=ControllerFunc  OutputSignalType=real
  W Data : MATLABFcn  MATLABFcn=LookupTable  OutputSignalType=real
  W ID : Constant  Value=9
  grid Controller : MATLABFcn  MATLABFcn=ControllerFunc  OutputSignalType=real
  p{1,15..17} (4 alike) : Product
  total consump : Outport
  total storage : Outport  Port=2
  total grid : Outport  Port=3
  wires:
  Clock1/1 -> Mux10/3, Mux14/3, Scope/5, Consumer Scope/2  "time"
  W Data/1 -> p1/1
  Solar Data/1 -> Gain4/1
  Solar Controller/1 -> p15/2
  Gain10/1 -> Scope/2, Mux1/1, p15/1  "Solar"
  p15/1 -> Sum/1, Scope/1  "Solar out"
  Sum/1 -> p16/1
  Battery Controller/1 -> p16/2
  Sum1/1 -> total storage/1, Scope/3  "Battery charge"
  grid Controller/1 -> p17/2
  p17/1 -> Scope/6, total grid/1  "grid input"
  Read Batery Charge/1 -> Sum1/1, Mux1/2
  p16/1 -> Mux1/3  "Battery in"
  ProcessBatteryOut/1 -> Scope/4, Sum1/2  "Battery in"
  Mux1/1 -> ProcessBatteryOut/1
  Gain4/1 -> Gain10/1
  W ID/1 -> Mux2/1, Mux10/2
  House ID/1 -> Mux10/1, Mux14/1
  Mux6/1 -> Solar Controller/1
  Solar ID/1 -> Mux14/2, Mux6/1
  Mux7/1 -> Battery Controller/1
  Mux8/1 -> Read Batery Charge/1
  Mux9/1 -> grid Controller/1
  Battery ID/1 -> Mux7/1
  Battery Charge ID/1 -> Mux8/1
  Grid ID/1 -> Mux9/1
  Mux10/1 -> W Data/1
  Mux14/1 -> Solar Data/1
  W Controller/1 -> p1/2
  Mux2/1 -> W Controller/1
  p1/1 -> p17/1, Sum/2, total consump/1, Consumer Scope/1  "consumption"
  House CommandID/1 -> Mux9/2, Mux8/2, Mux7/2, Mux6/2, Mux2/2

== system a4/House 4R5 ==
  House ID : Inport
  House CommandID : Inport  Port=2
  Battery Charge ID : Constant  Value=2
  Battery Controller : MATLABFcn  MATLABFcn=ControllerFunc  OutputSignalType=real
  Battery ID : Constant  Value=3
  Clock1 : Clock
  Consumer Scope : Scope  NumInputPorts=2
  Gain10 : Gain  Gain=sqrt(2)
  Gain4 : Gain  Gain=1/20
  Grid ID : Constant
  Mux1 : Mux  Inputs=3
  Mux10 : Mux  Inputs=3
  Mux14 : Mux  Inputs=3
  Mux{2,6..9} (5 alike) : Mux  Inputs=2
  ProcessBatteryOut : MATLABFcn  MATLABFcn=ProcessBatteryOutWFunc  OutputSignalType=real
  Read Batery Charge : MATLABFcn  MATLABFcn=ControllerFunc  OutputSignalType=real
  Scope : Scope  NumInputPorts=6
  Solar Controller : MATLABFcn  MATLABFcn=ControllerFunc  OutputSignalType=real
  Solar Data : MATLABFcn  MATLABFcn=LookupTable  OutputSignalType=real
  Solar ID : Constant  Value=4
  Sum : Sum  Inputs=|+-
  Sum1 : Sum  Inputs=|++
  W Controller : MATLABFcn  MATLABFcn=ControllerFunc  OutputSignalType=real
  W Data : MATLABFcn  MATLABFcn=LookupTable  OutputSignalType=real
  W ID : Constant  Value=9
  grid Controller : MATLABFcn  MATLABFcn=ControllerFunc  OutputSignalType=real
  p{1,15..17} (4 alike) : Product
  total consump : Outport
  total storage : Outport  Port=2
  total grid : Outport  Port=3
  wires:
  House CommandID/1 -> Mux2/2, Mux6/2, Mux7/2, Mux8/2, Mux9/2
  p1/1 -> Consumer Scope/1, total consump/1, Sum/2, p17/1  "consumption"
  Mux2/1 -> W Controller/1
  W Controller/1 -> p1/2
  Mux14/1 -> Solar Data/1
  Mux10/1 -> W Data/1
  Grid ID/1 -> Mux9/1
  Battery Charge ID/1 -> Mux8/1
  Battery ID/1 -> Mux7/1
  Mux9/1 -> grid Controller/1
  Mux8/1 -> Read Batery Charge/1
  Mux7/1 -> Battery Controller/1
  Solar ID/1 -> Mux6/1, Mux14/2
  Mux6/1 -> Solar Controller/1
  House ID/1 -> Mux14/1, Mux10/1
  W ID/1 -> Mux10/2, Mux2/1
  Gain4/1 -> Gain10/1
  Mux1/1 -> ProcessBatteryOut/1
  ProcessBatteryOut/1 -> Sum1/2, Scope/4  "Battery in"
  p16/1 -> Mux1/3  "Battery in"
  Read Batery Charge/1 -> Mux1/2, Sum1/1
  p17/1 -> total grid/1, Scope/6  "grid input"
  grid Controller/1 -> p17/2
  Sum1/1 -> Scope/3, total storage/1  "Battery charge"
  Battery Controller/1 -> p16/2
  Sum/1 -> p16/1
  p15/1 -> Scope/1, Sum/1  "Solar out"
  Gain10/1 -> p15/1, Mux1/1, Scope/2  "Solar"
  Solar Controller/1 -> p15/2
  Solar Data/1 -> Gain4/1
  W Data/1 -> p1/1
  Clock1/1 -> Consumer Scope/2, Scope/5, Mux14/3, Mux10/3  "time"

== system a4/House 5R1 ==
  House ID : Inport
  House CommandID : Inport  Port=2
  Battery Charge ID : Constant  Value=2
  Battery Controller : MATLABFcn  MATLABFcn=ControllerFunc  OutputSignalType=real
  Battery ID : Constant  Value=3
  Clock1 : Clock
  Consumer Scope : Scope  NumInputPorts=2
  Gain10 : Gain  Gain=sqrt(2)
  Gain4 : Gain  Gain=1/20
  Grid ID : Constant
  Mux1 : Mux  Inputs=3
  Mux10 : Mux  Inputs=3
  Mux14 : Mux  Inputs=3
  Mux{2,6..9} (5 alike) : Mux  Inputs=2
  ProcessBatteryOut : MATLABFcn  MATLABFcn=ProcessBatteryOutWFunc  OutputSignalType=real
  Read Batery Charge : MATLABFcn  MATLABFcn=ControllerFunc  OutputSignalType=real
  Scope : Scope  NumInputPorts=6
  Solar Controller : MATLABFcn  MATLABFcn=ControllerFunc  OutputSignalType=real
  Solar Data : MATLABFcn  MATLABFcn=LookupTable  OutputSignalType=real
  Solar ID : Constant  Value=4
  Sum : Sum  Inputs=|+-
  Sum1 : Sum  Inputs=|++
  W Controller : MATLABFcn  MATLABFcn=ControllerFunc  OutputSignalType=real
  W Data : MATLABFcn  MATLABFcn=LookupTable  OutputSignalType=real
  W ID : Constant  Value=9
  grid Controller : MATLABFcn  MATLABFcn=ControllerFunc  OutputSignalType=real
  p{1,15..17} (4 alike) : Product
  total consump : Outport
  total storage : Outport  Port=2
  total grid : Outport  Port=3
  wires:
  Clock1/1 -> Mux10/3, Mux14/3, Scope/5, Consumer Scope/2  "time"
  W Data/1 -> p1/1
  Solar Data/1 -> Gain4/1
  Solar Controller/1 -> p15/2
  Gain10/1 -> Scope/2, Mux1/1, p15/1  "Solar"
  p15/1 -> Sum/1, Scope/1  "Solar out"
  Sum/1 -> p16/1
  Battery Controller/1 -> p16/2
  Sum1/1 -> total storage/1, Scope/3  "Battery charge"
  grid Controller/1 -> p17/2
  p17/1 -> Scope/6, total grid/1  "grid input"
  Read Batery Charge/1 -> Sum1/1, Mux1/2
  p16/1 -> Mux1/3  "Battery in"
  ProcessBatteryOut/1 -> Scope/4, Sum1/2  "Battery in"
  Mux1/1 -> ProcessBatteryOut/1
  Gain4/1 -> Gain10/1
  W ID/1 -> Mux2/1, Mux10/2
  House ID/1 -> Mux10/1, Mux14/1
  Mux6/1 -> Solar Controller/1
  Solar ID/1 -> Mux14/2, Mux6/1
  Mux7/1 -> Battery Controller/1
  Mux8/1 -> Read Batery Charge/1
  Mux9/1 -> grid Controller/1
  Battery ID/1 -> Mux7/1
  Battery Charge ID/1 -> Mux8/1
  Grid ID/1 -> Mux9/1
  Mux10/1 -> W Data/1
  Mux14/1 -> Solar Data/1
  W Controller/1 -> p1/2
  Mux2/1 -> W Controller/1
  p1/1 -> p17/1, Sum/2, total consump/1, Consumer Scope/1  "consumption"
  House CommandID/1 -> Mux9/2, Mux8/2, Mux7/2, Mux6/2, Mux2/2

== system a4/House 5R2 ==
  House ID : Inport
  House CommandID : Inport  Port=2
  Battery Charge ID : Constant  Value=2
  Battery Controller : MATLABFcn  MATLABFcn=ControllerFunc  OutputSignalType=real
  Battery ID : Constant  Value=3
  Clock1 : Clock
  Consumer Scope : Scope  NumInputPorts=2
  Gain10 : Gain  Gain=sqrt(2)
  Gain4 : Gain  Gain=1/20
  Grid ID : Constant
  Mux1 : Mux  Inputs=3
  Mux10 : Mux  Inputs=3
  Mux14 : Mux  Inputs=3
  Mux{2,6..9} (5 alike) : Mux  Inputs=2
  ProcessBatteryOut : MATLABFcn  MATLABFcn=ProcessBatteryOutWFunc  OutputSignalType=real
  Read Batery Charge : MATLABFcn  MATLABFcn=ControllerFunc  OutputSignalType=real
  Scope : Scope  NumInputPorts=6
  Solar Controller : MATLABFcn  MATLABFcn=ControllerFunc  OutputSignalType=real
  Solar Data : MATLABFcn  MATLABFcn=LookupTable  OutputSignalType=real
  Solar ID : Constant  Value=4
  Sum : Sum  Inputs=|+-
  Sum1 : Sum  Inputs=|++
  W Controller : MATLABFcn  MATLABFcn=ControllerFunc  OutputSignalType=real
  W Data : MATLABFcn  MATLABFcn=LookupTable  OutputSignalType=real
  W ID : Constant  Value=9
  grid Controller : MATLABFcn  MATLABFcn=ControllerFunc  OutputSignalType=real
  p{1,15..17} (4 alike) : Product
  total consump : Outport
  total storage : Outport  Port=2
  total grid : Outport  Port=3
  wires:
  House CommandID/1 -> Mux2/2, Mux6/2, Mux7/2, Mux8/2, Mux9/2
  p1/1 -> Consumer Scope/1, total consump/1, Sum/2, p17/1  "consumption"
  Mux2/1 -> W Controller/1
  W Controller/1 -> p1/2
  Mux14/1 -> Solar Data/1
  Mux10/1 -> W Data/1
  Grid ID/1 -> Mux9/1
  Battery Charge ID/1 -> Mux8/1
  Battery ID/1 -> Mux7/1
  Mux9/1 -> grid Controller/1
  Mux8/1 -> Read Batery Charge/1
  Mux7/1 -> Battery Controller/1
  Solar ID/1 -> Mux6/1, Mux14/2
  Mux6/1 -> Solar Controller/1
  House ID/1 -> Mux14/1, Mux10/1
  W ID/1 -> Mux10/2, Mux2/1
  Gain4/1 -> Gain10/1
  Mux1/1 -> ProcessBatteryOut/1
  ProcessBatteryOut/1 -> Sum1/2, Scope/4  "Battery in"
  p16/1 -> Mux1/3  "Battery in"
  Read Batery Charge/1 -> Mux1/2, Sum1/1
  p17/1 -> total grid/1, Scope/6  "grid input"
  grid Controller/1 -> p17/2
  Sum1/1 -> Scope/3, total storage/1  "Battery charge"
  Battery Controller/1 -> p16/2
  Sum/1 -> p16/1
  p15/1 -> Scope/1, Sum/1  "Solar out"
  Gain10/1 -> p15/1, Mux1/1, Scope/2  "Solar"
  Solar Controller/1 -> p15/2
  Solar Data/1 -> Gain4/1
  W Data/1 -> p1/1
  Clock1/1 -> Consumer Scope/2, Scope/5, Mux14/3, Mux10/3  "time"

== system a4/House 5R3 ==
  House ID : Inport
  House CommandID : Inport  Port=2
  Battery Charge ID : Constant  Value=2
  Battery Controller : MATLABFcn  MATLABFcn=ControllerFunc  OutputSignalType=real
  Battery ID : Constant  Value=3
  Clock1 : Clock
  Consumer Scope : Scope  NumInputPorts=2
  Gain10 : Gain  Gain=sqrt(2)
  Gain4 : Gain  Gain=1/20
  Grid ID : Constant
  Mux1 : Mux  Inputs=3
  Mux10 : Mux  Inputs=3
  Mux14 : Mux  Inputs=3
  Mux{2,6..9} (5 alike) : Mux  Inputs=2
  ProcessBatteryOut : MATLABFcn  MATLABFcn=ProcessBatteryOutWFunc  OutputSignalType=real
  Read Batery Charge : MATLABFcn  MATLABFcn=ControllerFunc  OutputSignalType=real
  Scope : Scope  NumInputPorts=6
  Solar Controller : MATLABFcn  MATLABFcn=ControllerFunc  OutputSignalType=real
  Solar Data : MATLABFcn  MATLABFcn=LookupTable  OutputSignalType=real
  Solar ID : Constant  Value=4
  Sum : Sum  Inputs=|+-
  Sum1 : Sum  Inputs=|++
  W Controller : MATLABFcn  MATLABFcn=ControllerFunc  OutputSignalType=real
  W Data : MATLABFcn  MATLABFcn=LookupTable  OutputSignalType=real
  W ID : Constant  Value=9
  grid Controller : MATLABFcn  MATLABFcn=ControllerFunc  OutputSignalType=real
  p{1,15..17} (4 alike) : Product
  total consump : Outport
  total storage : Outport  Port=2
  total grid : Outport  Port=3
  wires:
  Clock1/1 -> Mux10/3, Mux14/3, Scope/5, Consumer Scope/2  "time"
  W Data/1 -> p1/1
  Solar Data/1 -> Gain4/1
  Solar Controller/1 -> p15/2
  Gain10/1 -> Scope/2, Mux1/1, p15/1  "Solar"
  p15/1 -> Sum/1, Scope/1  "Solar out"
  Sum/1 -> p16/1
  Battery Controller/1 -> p16/2
  Sum1/1 -> total storage/1, Scope/3  "Battery charge"
  grid Controller/1 -> p17/2
  p17/1 -> Scope/6, total grid/1  "grid input"
  Read Batery Charge/1 -> Sum1/1, Mux1/2
  p16/1 -> Mux1/3  "Battery in"
  ProcessBatteryOut/1 -> Scope/4, Sum1/2  "Battery in"
  Mux1/1 -> ProcessBatteryOut/1
  Gain4/1 -> Gain10/1
  W ID/1 -> Mux2/1, Mux10/2
  House ID/1 -> Mux10/1, Mux14/1
  Mux6/1 -> Solar Controller/1
  Solar ID/1 -> Mux14/2, Mux6/1
  Mux7/1 -> Battery Controller/1
  Mux8/1 -> Read Batery Charge/1
  Mux9/1 -> grid Controller/1
  Battery ID/1 -> Mux7/1
  Battery Charge ID/1 -> Mux8/1
  Grid ID/1 -> Mux9/1
  Mux10/1 -> W Data/1
  Mux14/1 -> Solar Data/1
  W Controller/1 -> p1/2
  Mux2/1 -> W Controller/1
  p1/1 -> p17/1, Sum/2, total consump/1, Consumer Scope/1  "consumption"
  House CommandID/1 -> Mux9/2, Mux8/2, Mux7/2, Mux6/2, Mux2/2

== system a4/House 5R4 ==
  House ID : Inport
  House CommandID : Inport  Port=2
  Battery Charge ID : Constant  Value=2
  Battery Controller : MATLABFcn  MATLABFcn=ControllerFunc  OutputSignalType=real
  Battery ID : Constant  Value=3
  Clock1 : Clock
  Consumer Scope : Scope  NumInputPorts=2
  Gain10 : Gain  Gain=sqrt(2)
  Gain4 : Gain  Gain=1/20
  Grid ID : Constant
  Mux1 : Mux  Inputs=3
  Mux10 : Mux  Inputs=3
  Mux14 : Mux  Inputs=3
  Mux{2,6..9} (5 alike) : Mux  Inputs=2
  ProcessBatteryOut : MATLABFcn  MATLABFcn=ProcessBatteryOutWFunc  OutputSignalType=real
  Read Batery Charge : MATLABFcn  MATLABFcn=ControllerFunc  OutputSignalType=real
  Scope : Scope  NumInputPorts=6
  Solar Controller : MATLABFcn  MATLABFcn=ControllerFunc  OutputSignalType=real
  Solar Data : MATLABFcn  MATLABFcn=LookupTable  OutputSignalType=real
  Solar ID : Constant  Value=4
  Sum : Sum  Inputs=|+-
  Sum1 : Sum  Inputs=|++
  W Controller : MATLABFcn  MATLABFcn=ControllerFunc  OutputSignalType=real
  W Data : MATLABFcn  MATLABFcn=LookupTable  OutputSignalType=real
  W ID : Constant  Value=9
  grid Controller : MATLABFcn  MATLABFcn=ControllerFunc  OutputSignalType=real
  p{1,15..17} (4 alike) : Product
  total consump : Outport
  total storage : Outport  Port=2
  total grid : Outport  Port=3
  wires:
  House CommandID/1 -> Mux2/2, Mux6/2, Mux7/2, Mux8/2, Mux9/2
  p1/1 -> Consumer Scope/1, total consump/1, Sum/2, p17/1  "consumption"
  Mux2/1 -> W Controller/1
  W Controller/1 -> p1/2
  Mux14/1 -> Solar Data/1
  Mux10/1 -> W Data/1
  Grid ID/1 -> Mux9/1
  Battery Charge ID/1 -> Mux8/1
  Battery ID/1 -> Mux7/1
  Mux9/1 -> grid Controller/1
  Mux8/1 -> Read Batery Charge/1
  Mux7/1 -> Battery Controller/1
  Solar ID/1 -> Mux6/1, Mux14/2
  Mux6/1 -> Solar Controller/1
  House ID/1 -> Mux14/1, Mux10/1
  W ID/1 -> Mux10/2, Mux2/1
  Gain4/1 -> Gain10/1
  Mux1/1 -> ProcessBatteryOut/1
  ProcessBatteryOut/1 -> Sum1/2, Scope/4  "Battery in"
  p16/1 -> Mux1/3  "Battery in"
  Read Batery Charge/1 -> Mux1/2, Sum1/1
  p17/1 -> total grid/1, Scope/6  "grid input"
  grid Controller/1 -> p17/2
  Sum1/1 -> Scope/3, total storage/1  "Battery charge"
  Battery Controller/1 -> p16/2
  Sum/1 -> p16/1
  p15/1 -> Scope/1, Sum/1  "Solar out"
  Gain10/1 -> p15/1, Mux1/1, Scope/2  "Solar"
  Solar Controller/1 -> p15/2
  Solar Data/1 -> Gain4/1
  W Data/1 -> p1/1
  Clock1/1 -> Consumer Scope/2, Scope/5, Mux14/3, Mux10/3  "time"

== system a4/House 5R5 ==
  House ID : Inport
  House CommandID : Inport  Port=2
  Battery Charge ID : Constant  Value=2
  Battery Controller : MATLABFcn  MATLABFcn=ControllerFunc  OutputSignalType=real
  Battery ID : Constant  Value=3
  Clock1 : Clock
  Consumer Scope : Scope  NumInputPorts=2
  Gain10 : Gain  Gain=sqrt(2)
  Gain4 : Gain  Gain=1/20
  Grid ID : Constant
  Mux1 : Mux  Inputs=3
  Mux10 : Mux  Inputs=3
  Mux14 : Mux  Inputs=3
  Mux{2,6..9} (5 alike) : Mux  Inputs=2
  ProcessBatteryOut : MATLABFcn  MATLABFcn=ProcessBatteryOutWFunc  OutputSignalType=real
  Read Batery Charge : MATLABFcn  MATLABFcn=ControllerFunc  OutputSignalType=real
  Scope : Scope  NumInputPorts=6
  Solar Controller : MATLABFcn  MATLABFcn=ControllerFunc  OutputSignalType=real
  Solar Data : MATLABFcn  MATLABFcn=LookupTable  OutputSignalType=real
  Solar ID : Constant  Value=4
  Sum : Sum  Inputs=|+-
  Sum1 : Sum  Inputs=|++
  W Controller : MATLABFcn  MATLABFcn=ControllerFunc  OutputSignalType=real
  W Data : MATLABFcn  MATLABFcn=LookupTable  OutputSignalType=real
  W ID : Constant  Value=9
  grid Controller : MATLABFcn  MATLABFcn=ControllerFunc  OutputSignalType=real
  p{1,15..17} (4 alike) : Product
  total consump : Outport
  total storage : Outport  Port=2
  total grid : Outport  Port=3
  wires:
  Clock1/1 -> Mux10/3, Mux14/3, Scope/5, Consumer Scope/2  "time"
  W Data/1 -> p1/1
  Solar Data/1 -> Gain4/1
  Solar Controller/1 -> p15/2
  Gain10/1 -> Scope/2, Mux1/1, p15/1  "Solar"
  p15/1 -> Sum/1, Scope/1  "Solar out"
  Sum/1 -> p16/1
  Battery Controller/1 -> p16/2
  Sum1/1 -> total storage/1, Scope/3  "Battery charge"
  grid Controller/1 -> p17/2
  p17/1 -> Scope/6, total grid/1  "grid input"
  Read Batery Charge/1 -> Sum1/1, Mux1/2
  p16/1 -> Mux1/3  "Battery in"
  ProcessBatteryOut/1 -> Scope/4, Sum1/2  "Battery in"
  Mux1/1 -> ProcessBatteryOut/1
  Gain4/1 -> Gain10/1
  W ID/1 -> Mux2/1, Mux10/2
  House ID/1 -> Mux10/1, Mux14/1
  Mux6/1 -> Solar Controller/1
  Solar ID/1 -> Mux14/2, Mux6/1
  Mux7/1 -> Battery Controller/1
  Mux8/1 -> Read Batery Charge/1
  Mux9/1 -> grid Controller/1
  Battery ID/1 -> Mux7/1
  Battery Charge ID/1 -> Mux8/1
  Grid ID/1 -> Mux9/1
  Mux10/1 -> W Data/1
  Mux14/1 -> Solar Data/1
  W Controller/1 -> p1/2
  Mux2/1 -> W Controller/1
  p1/1 -> p17/1, Sum/2, total consump/1, Consumer Scope/1  "consumption"
  House CommandID/1 -> Mux9/2, Mux8/2, Mux7/2, Mux6/2, Mux2/2
